simulink library "stimulation_staticAngles_lib"  (Simulink 6.2)
settings Model: LastModifiedBy=bsaunder  ExtModeAutoUpdateStatusClock=off

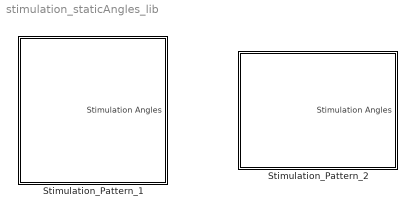
== system stimulation_staticAngles_lib ==
  Stimulation_Pattern_1 : Subsystem  mask(StimAnglesInput){Quad_R=[55 155], Ham_R=[188 265], Glut_R=[90 180], Calf_R=[180 205], ExactOpp=on, Quad_L=[235  335], Ham_L=[8  85], Glut_L=[270    0], Calf_L=[0  25]}
      mask prompts: Quad_R "Quad. Right"; Ham_R "Ham. Right"; Glut_R "Glut. Right"; Calf_R "Calf Right"; ExactOpp "Force left leg to be 180 degrees opposite from right leg"; Quad_L "Quad. Left"; Ham_L "Ham. Left"; Glut_L "Glut. Left"; Calf_L "Calf Left"
      mask help: Use this block to input the stimulation angles. Angles should be in degrees and be between 0 and 360. The format should be a 2 element vector to indicate the start and stop angles e.g. [start stop]. Output is a bus signal.
      mask init:
      | if ExactOpp
      |   Quad_L = Quad_R+180;
      |   Quad_L = Quad_L - 360*floor(Quad_L/360);
      |   set_param(gcb, 'Quad_L', ['[',num2str(Quad_L),']']);
      | 
      |   Ham_L = Ham_R+180;
      |   Ham_L = Ham_L - 360*floor(Ham_L/360);
      |   set_param(gcb, 'Ham_L', ['[',num2str(Ham_L),']']);
      | 
      |   Glut_L = Glut_R+180;
      |   Glut_L = Glut_L - 360*floor(Glut_L/360);
      |   set_param(gcb, 'Glut_L', ['[',num2str(Glut_L),']']);
      | 
      |   Calf_L = Calf_R+180;
      |   Calf_L = Calf_L - 360*floor(Calf_L/360);
      |   set_param(gcb, 'Calf_L', ['[',num2str(Calf_L),']']);
      | end
      | 
      | circle_center = [0.4, 0.4]; circle_radius = 0.35;
      | icon_circle_x = circle_radius.*sin([0:pi/18:2*pi]) + circle_center(1);
      | icon_circle_y = circle_radius.*cos([0:pi/18:2*pi]) + circle_center(2);
      | 
      | patch_width = 0.04;
      | ip_params = [...
      |     Quad_R(1), Quad_R(2), 0.34; ...
      |     Quad_L(1), Quad_L(2), 0.34; ...
      |     Ham_R(1),  Ham_R(2),  0.29; ...
      |     Ham_L(1),  Ham_L(2),  0.29; ...
      |     Glut_R(1), Glut_R(2), 0.24; ...
      |     Glut_L(1), Glut_L(2), 0.24; ...
      |     Calf_R(1), Calf_R(2), 0.19; ...
      |     Calf_L(1), Calf_L(2), 0.19; ...
      |     ];
      | 
      | ip_params(:,1) = ip_params(:,1)+90;
      | ip_params(:,2) = ip_params(:,2)+90;
      | 
      | for i = 1 : length(ip_params(:,1))
      |     if ip_params(i,2) < ip_params(i,1) ip_params(i,2) = ip_params(i,2) + 360; end
      |     x_outer = ip_params(i,3).*sin([(ip_params(i,1)/180)*pi:pi/18:(ip_params(i,2)/180)*pi]) + circle_center(1);
      |     y_outer = ip_params(i,3).*cos([(ip_params(i,1)/180)*pi:pi/18:(ip_params(i,2)/180)*pi]) + circle_center(1);
      |     x_inner = (ip_params(i,3)-patch_width).*sin([(ip_params(i,2)/180)*pi:-pi/18:(ip_params(i,1)/180)*pi]) + circle_center(1);
      |     y_inner = (ip_params(i,3)-patch_width).*cos([(ip_params(i,2)/180)*pi:-pi/18:(ip_params(i,1)/180)*pi]) + circle_center(1);
      |     patch_coord_x{i} = [x_outer x_inner];
      |     patch_coord_y{i} = [y_outer y_inner];
      | end
      mask CallbackString:
      | ||||if strcmp(get_param(gcb,'ExactOpp'),'on')
      | set_param(gcb,'MaskVisibilities', {'on', 'on', 'on', 'on', 'on', 'off', 'off', 'off', 'off'});
      | else
      | set_param(gcb,'MaskVisibilities', {'on', 'on', 'on', 'on', 'on', 'on', 'on', 'on', 'on'});
      | end
      | ||||
      mask Display:
      | text(0.5, 0.9, 'Static Stimulation Angles', 'HorizontalAlignment', 'center', 'VerticalAlignment', 'middle');
      | 
      | plot(icon_circle_x, icon_circle_y);
      | patch(patch_coord_x{1}, patch_coord_y{1}, [1 0 0]);
      | patch(patch_coord_x{2}, patch_coord_y{2}, [1 0 0]);
      | patch(patch_coord_x{3}, patch_coord_y{3}, [0 0 1]);
      | patch(patch_coord_x{4}, patch_coord_y{4}, [0 0 1]);
      | patch(patch_coord_x{5}, patch_coord_y{5}, [0 1 0]);
      | patch(patch_coord_x{6}, patch_coord_y{6}, [0 1 0]);
      | patch(patch_coord_x{7}, patch_coord_y{7}, [0.8 0.8 0]);
      | patch(patch_coord_x{8}, patch_coord_y{8}, [0.8 0.8 0]);
      | 
      | plot(circle_center(1)+[0 circle_radius+0.05], [circle_center(2) circle_center(2)]);
      | 
      | patch([0 -0.05 -0.05 0]+0.9, [-0.025 -0.025 0.025 0.025]+0.55, [1 0 0]);
      | text(0.92, 0.55, 'Q', 'HorizontalAlignment', 'left', 'VerticalAlignment', 'middle');
      | 
      | patch([0 -0.05 -0.05 0]+0.9, [-0.025 -0.025 0.025 0.025]+0.45, [0 0 1]);
      | text(0.92, 0.45, 'H', 'HorizontalAlignment', 'left', 'VerticalAlignment', 'middle');
      | 
      | patch([0 -0.05 -0.05 0]+0.9, [-0.025 -0.025 0.025 0.025]+0.35, [0 1 0]);
      | text(0.92, 0.35, 'G', 'HorizontalAlignment', 'left', 'VerticalAlignment', 'middle');
      | 
      | patch([0 -0.05 -0.05 0]+0.9, [-0.025 -0.025 0.025 0.025]+0.25, [0.8 0.8 0]);
      | text(0.92, 0.25, 'C', 'HorizontalAlignment', 'left', 'VerticalAlignment', 'middle');
  Stimulation_Pattern_2 : Subsystem  mask(StimAnglesInput){Quad_R=[55 155], Ham_R=[188 265], Glut_R=[90 180], Calf_R=[0 1], ExactOpp=on, Quad_L=[235  335], Ham_L=[8  85], Glut_L=[270    0], Calf_L=[180  181]}
      mask prompts: Quad_R "Quad. Right"; Ham_R "Ham. Right"; Glut_R "Glut. Right"; Calf_R "Calf Right"; ExactOpp "Force left leg to be 180 degrees opposite from right leg"; Quad_L "Quad. Left"; Ham_L "Ham. Left"; Glut_L "Glut. Left"; Calf_L "Calf Left"
      mask help: Use this block to input the stimulation angles. Angles should be in degrees and be between 0 and 360. The format should be a 2 element vector to indicate the start and stop angles e.g. [start stop]. Output is a bus signal.
      mask init:
      | if ExactOpp
      |   Quad_L = Quad_R+180;
      |   Quad_L = Quad_L - 360*floor(Quad_L/360);
      |   set_param(gcb, 'Quad_L', ['[',num2str(Quad_L),']']);
      | 
      |   Ham_L = Ham_R+180;
      |   Ham_L = Ham_L - 360*floor(Ham_L/360);
      |   set_param(gcb, 'Ham_L', ['[',num2str(Ham_L),']']);
      | 
      |   Glut_L = Glut_R+180;
      |   Glut_L = Glut_L - 360*floor(Glut_L/360);
      |   set_param(gcb, 'Glut_L', ['[',num2str(Glut_L),']']);
      | 
      |   Calf_L = Calf_R+180;
      |   Calf_L = Calf_L - 360*floor(Calf_L/360);
      |   set_param(gcb, 'Calf_L', ['[',num2str(Calf_L),']']);
      | end
      mask CallbackString:
      | ||||if strcmp(get_param(gcb,'ExactOpp'),'on')
      | set_param(gcb,'MaskVisibilities', {'on', 'on', 'on', 'on', 'on', 'off', 'off', 'off', 'off'});
      | else
      | set_param(gcb,'MaskVisibilities', {'on', 'on', 'on', 'on', 'on', 'on', 'on', 'on', 'on'});
      | end
      | ||||
      mask Display:
      | text(0.5, 0.9, 'Static Stimulation Angles', 'HorizontalAlignment', 'center', 'VerticalAlignment', 'middle');
      | 
      | plot([0.05 0.95], [0.65 0.65]);
      | plot([0.2 0.2], [0.8 0.2]);
      | plot([0.6 0.6], [0.8 0.2]);
      | 
      | text(0.1, 0.7, 'M', 'HorizontalAlignment', 'center', 'VerticalAlignment', 'middle');
      | text(0.4, 0.7, 'Right', 'HorizontalAlignment', 'center', 'VerticalAlignment', 'middle');
      | text(0.8, 0.7, 'Left', 'HorizontalAlignment', 'center', 'VerticalAlignment', 'middle');
      | 
      | text(0.1, 0.55, 'Q', 'HorizontalAlignment', 'center', 'VerticalAlignment', 'middle');
      | text(0.4, 0.55, num2str(Quad_R), 'HorizontalAlignment', 'center', 'VerticalAlignment', 'middle');
      | text(0.8, 0.55, num2str(Quad_L), 'HorizontalAlignment', 'center', 'VerticalAlignment', 'middle');
      | 
      | text(0.1, 0.45, 'H', 'HorizontalAlignment', 'center', 'VerticalAlignment', 'middle');
      | text(0.4, 0.45, num2str(Ham_R), 'HorizontalAlignment', 'center', 'VerticalAlignment', 'middle');
      | text(0.8, 0.45, num2str(Ham_L), 'HorizontalAlignment', 'center', 'VerticalAlignment', 'middle');
      | 
      | text(0.1, 0.35, 'G', 'HorizontalAlignment', 'center', 'VerticalAlignment', 'middle');
      | text(0.4, 0.35, num2str(Glut_R), 'HorizontalAlignment', 'center', 'VerticalAlignment', 'middle');
      | text(0.8, 0.35, num2str(Glut_L), 'HorizontalAlignment', 'center', 'VerticalAlignment', 'middle');
      | 
      | text(0.1, 0.25, 'C', 'HorizontalAlignment', 'center', 'VerticalAlignment', 'middle');
      | text(0.4, 0.25, num2str(Calf_R), 'HorizontalAlignment', 'center', 'VerticalAlignment', 'middle');
      | text(0.8, 0.25, num2str(Calf_L), 'HorizontalAlignment', 'center', 'VerticalAlignment', 'middle');

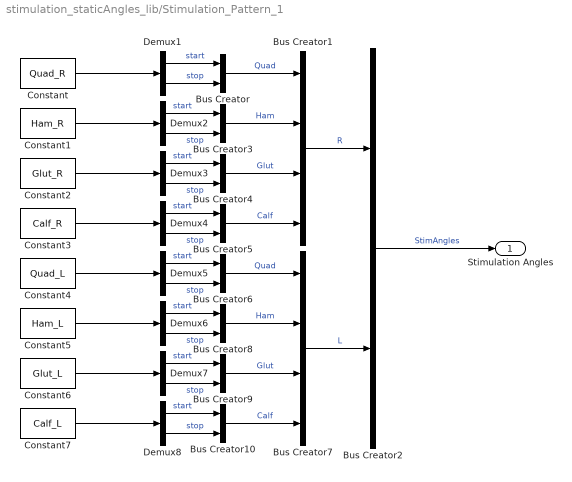
== system stimulation_staticAngles_lib/Stimulation_Pattern_1 ==
  Bus Creator{,2..6,8..10} (9 alike) : BusCreator  Inputs=2
  Bus Creator1 : BusCreator
  Bus Creator7 : BusCreator
  Constant : Constant  Value=Quad_R
  Constant1 : Constant  Value=Ham_R
  Constant2 : Constant  Value=Glut_R
  Constant3 : Constant  Value=Calf_R
  Constant4 : Constant  Value=Quad_L
  Constant5 : Constant  Value=Ham_L
  Constant6 : Constant  Value=Glut_L
  Constant7 : Constant  Value=Calf_L
  Demux{1..8} (8 alike) : Demux  Outputs=2
  Stimulation Angles : Outport
  wires:
  Bus Creator7/1 -> Bus Creator2/2  "L"
  Constant7/1 -> Demux8/1
  Constant6/1 -> Demux7/1
  Constant5/1 -> Demux6/1
  Constant4/1 -> Demux5/1
  Bus Creator10/1 -> Bus Creator7/4  "Calf"
  Bus Creator9/1 -> Bus Creator7/3  "Glut"
  Bus Creator8/1 -> Bus Creator7/2  "Ham"
  Demux8/2 -> Bus Creator10/2  "stop"
  Demux8/1 -> Bus Creator10/1  "start"
  Demux7/2 -> Bus Creator9/2  "stop"
  Demux7/1 -> Bus Creator9/1  "start"
  Demux6/2 -> Bus Creator8/2  "stop"
  Demux6/1 -> Bus Creator8/1  "start"
  Bus Creator6/1 -> Bus Creator7/1  "Quad"
  Demux5/2 -> Bus Creator6/2  "stop"
  Demux5/1 -> Bus Creator6/1  "start"
  Constant3/1 -> Demux4/1
  Constant2/1 -> Demux3/1
  Constant1/1 -> Demux2/1
  Bus Creator5/1 -> Bus Creator1/4  "Calf"
  Bus Creator4/1 -> Bus Creator1/3  "Glut"
  Bus Creator3/1 -> Bus Creator1/2  "Ham"
  Demux4/2 -> Bus Creator5/2  "stop"
  Demux4/1 -> Bus Creator5/1  "start"
  Demux3/2 -> Bus Creator4/2  "stop"
  Demux3/1 -> Bus Creator4/1  "start"
  Demux2/2 -> Bus Creator3/2  "stop"
  Demux2/1 -> Bus Creator3/1  "start"
  Bus Creator2/1 -> Stimulation Angles/1  "StimAngles"
  Bus Creator1/1 -> Bus Creator2/1  "R"
  Bus Creator/1 -> Bus Creator1/1  "Quad"
  Demux1/2 -> Bus Creator/2  "stop"
  Demux1/1 -> Bus Creator/1  "start"
  Constant/1 -> Demux1/1

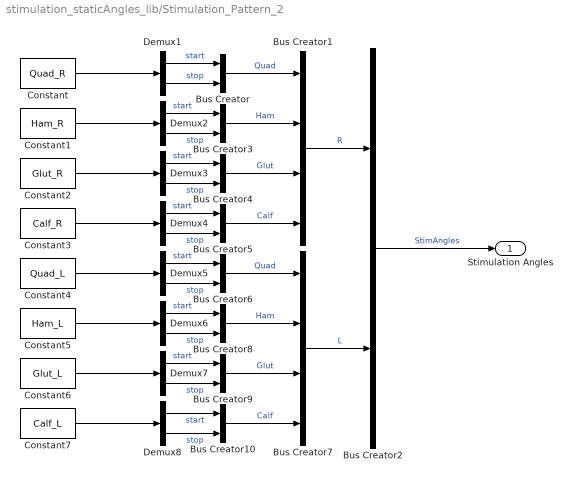
== system stimulation_staticAngles_lib/Stimulation_Pattern_2 ==
  Bus Creator{,2..6,8..10} (9 alike) : BusCreator  Inputs=2
  Bus Creator1 : BusCreator
  Bus Creator7 : BusCreator
  Constant : Constant  Value=Quad_R
  Constant1 : Constant  Value=Ham_R
  Constant2 : Constant  Value=Glut_R
  Constant3 : Constant  Value=Calf_R
  Constant4 : Constant  Value=Quad_L
  Constant5 : Constant  Value=Ham_L
  Constant6 : Constant  Value=Glut_L
  Constant7 : Constant  Value=Calf_L
  Demux{1..8} (8 alike) : Demux  Outputs=2
  Stimulation Angles : Outport
  wires:
  Constant/1 -> Demux1/1
  Demux1/1 -> Bus Creator/1  "start"
  Demux1/2 -> Bus Creator/2  "stop"
  Bus Creator/1 -> Bus Creator1/1  "Quad"
  Bus Creator1/1 -> Bus Creator2/1  "R"
  Bus Creator2/1 -> Stimulation Angles/1  "StimAngles"
  Demux2/1 -> Bus Creator3/1  "start"
  Demux2/2 -> Bus Creator3/2  "stop"
  Demux3/1 -> Bus Creator4/1  "start"
  Demux3/2 -> Bus Creator4/2  "stop"
  Demux4/1 -> Bus Creator5/1  "start"
  Demux4/2 -> Bus Creator5/2  "stop"
  Bus Creator3/1 -> Bus Creator1/2  "Ham"
  Bus Creator4/1 -> Bus Creator1/3  "Glut"
  Bus Creator5/1 -> Bus Creator1/4  "Calf"
  Constant1/1 -> Demux2/1
  Constant2/1 -> Demux3/1
  Constant3/1 -> Demux4/1
  Demux5/1 -> Bus Creator6/1  "start"
  Demux5/2 -> Bus Creator6/2  "stop"
  Bus Creator6/1 -> Bus Creator7/1  "Quad"
  Demux6/1 -> Bus Creator8/1  "start"
  Demux6/2 -> Bus Creator8/2  "stop"
  Demux7/1 -> Bus Creator9/1  "start"
  Demux7/2 -> Bus Creator9/2  "stop"
  Demux8/1 -> Bus Creator10/1  "start"
  Demux8/2 -> Bus Creator10/2  "stop"
  Bus Creator8/1 -> Bus Creator7/2  "Ham"
  Bus Creator9/1 -> Bus Creator7/3  "Glut"
  Bus Creator10/1 -> Bus Creator7/4  "Calf"
  Constant4/1 -> Demux5/1
  Constant5/1 -> Demux6/1
  Constant6/1 -> Demux7/1
  Constant7/1 -> Demux8/1
  Bus Creator7/1 -> Bus Creator2/2  "L"
